simulink model "BuckBoost_real"  (R2015b)
settings: Solver=VariableStepAuto  StartTime=0.0  StopTime=0.01  RelTol=0.001
values from neighbouring files (symbols this model uses):
  Rload = 10    [BuckBoost_script.m]
libraries: fl_lib x7, elec_lib x5, nesl_utility x5
settings Model: Creator=lukaskiechle  LastModifiedBy=lukaskiechle
settings DataIOCC: LimitDataPoints=off  SaveFormat=Array
settings DebuggingCC: MaxConsecutiveZCsMsg=none
settings SimscapeCC: SimscapeLogType=all  SimscapeLogSimulationStatistics=on  SimscapeLogOpenViewer=on

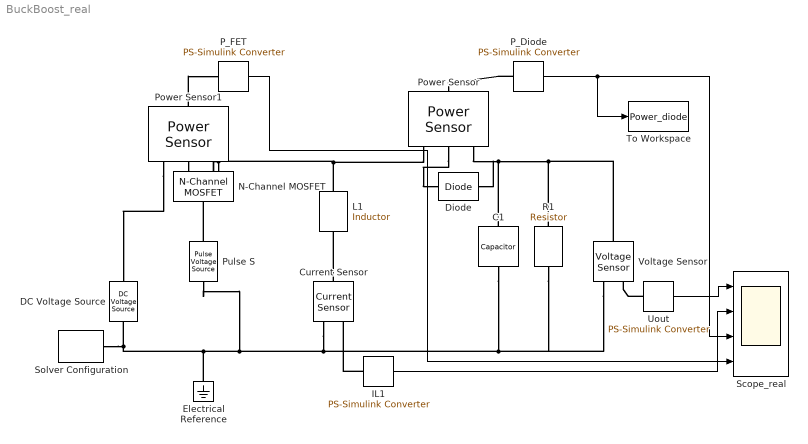
== system BuckBoost_real ==
  C1 : fl_lib/Electrical/Electrical Elements/Capacitor  c=C1 F  r=1e-9 Ohm  g=0 1/Ohm  i_specify=off  i_priority=None  i=0 A  v_specify=off  v_priority=None  v=0 V  vc_specify=off  vc_priority=None  vc=0 V
  Current Sensor : fl_lib/Electrical/Electrical Sensors/Current Sensor
  DC Voltage Source : fl_lib/Electrical/Electrical Sources/DC Voltage Source  v0=Uin V
  Diode : elec_lib/Semiconductor Devices/Diode  ModelType=2  Vf=UF V  Ron=0.08 Ohm  Goff=1E-9 S  Rz=0.1 Ohm  Vz=75 V  C_PWL=Diode_C F  prmExp=2  I12=[ 0.0137 0.545 ] A  V12=[ 0.6 0.7 ] V  I1=0.0137 A  V1=0.6 V  RS=0.01 Ohm  IS=1e-12 A  Tmeas=25 C  ec=1  BV=Inf V  C_param=1  CJ0=5 pF  VJ=1 V  Mgrad=0.5  Vvec=[ 0.1 10 100 ] V  Cvec=[ 3.5 1 0.4 ] pF  FC=0.5  Q_param=1  Irrm=-7.15 A  iF=4 A  didt=-750 A/us  trr=115 ns  TT=50 ns  tau=100 ns  T_param=1  IS_T2=1.25e-7 A  I1_T2=0.245 A  V1_T2=0.5 V  Tmeas2=125 C  EG_param=1  EG=1.11 eV  XTI_param=1  XTI=3  dBVdT=0 V/K  Tdevice=25 C  Rth=[ 0 10 ] K/W  thermal_mass_parameterization=1  thermal_mass=[ 0 1 ] J/K  thermal_time_constant=[ 0 10 ] s  thermal_mass_initial_temperatures=[ 25 25 ] C
  Electrical Reference : fl_lib/Electrical/Electrical Elements/Electrical Reference
  IL1 : nesl_utility/PS-Simulink Converter  PhysicalDomain=network_engine_domain  SubClassName=ps_output  LeftPortType=input  RightPortType=output  PseudoPeriodic=off  Frequencies=[]  Unit=A  AffineConversion=off
  L1 : fl_lib/Electrical/Electrical Elements/Inductor  l=L1 H  r=1 Ohm  g=1e-9 1/Ohm  i_specify=off  i_priority=None  i=0 A  v_specify=off  v_priority=None  v=0 V  i_L_specify=off  i_L_priority=None  i_L=0 A
  N-Channel MOSFET : elec_lib/Semiconductor Devices/N-Channel MOSFET  parameterization=1  prmDatasheet=1  prmEquCoeff=1  Beta=5 A/V^2  Rds=0.16 Ohm  Id=14 A  Vgs=10 V  Vth=3 V  lam=0 1/V  Tmeas=25 C  RS=1e-4 Ohm  RD=0.01 Ohm  C_param=1  C_GS=270 pF  C_GD=80 pF  C_iss=350 pF  C_rss=80 pF  C_oss=0 pF  C_GS_vec=[ 270 300 290 280 295 255 ] pF  C_GD_vec=[ 450 400 300 190 95 55 ] pF  C_iss_vec=[ 720 700 590 470 390 310 ] pF  C_rss_vec=[ 450 400 300 190 95 55 ] pF  C_oss_vec=[ 900 810 690 420 270 170 ] pF  C_Vds_vec=[ 0.1 0.3 1 3 10 30 ] V  charge_linearity_param=1  C_OX=200 pF  V_C_OX=-0.5 V  dVth_dT=-6 mV/K  Rds_T2=0.037 Ohm  Tmeas2=125 C  BEXDatasheet=-1.5  BEXEquCoeff=-1.5  TdeviceDatasheet=25 C  TdeviceEquCoeff=25 C  Rth=[ 0 10 ] K/W  thermal_mass_parameterization=1  thermal_mass=[ 0 1 ] J/K  thermal_time_constant=[ 0 10 ] s  thermal_mass_initial_temperatures=[ 25 25 ] C
  P_Diode : nesl_utility/PS-Simulink Converter  PhysicalDomain=network_engine_domain  SubClassName=ps_output  LeftPortType=input  RightPortType=output  PseudoPeriodic=off  Frequencies=[]  Unit=W  AffineConversion=off
  P_FET : nesl_utility/PS-Simulink Converter  PhysicalDomain=network_engine_domain  SubClassName=ps_output  LeftPortType=input  RightPortType=output  PseudoPeriodic=off  Frequencies=[]  Unit=W  AffineConversion=off
  Power Sensor : elec_lib/Sensors/Power Sensor  measurement_type=1  averaging_period=1 ms
  Power Sensor1 : elec_lib/Sensors/Power Sensor  measurement_type=1  averaging_period=1e-4 s
  Pulse S : elec_lib/Additional Components/SPICE-Compatible Components/Sources/Pulse Voltage Source  V1=0 V  V2=Upulse V  TD=0 s  TR=1e-9 s  TF=1e-9 s  PW=Ton s  PER=Twidth s
  R1 : fl_lib/Electrical/Electrical Elements/Resistor  R=Rload Ohm  i_specify=off  i_priority=None  i=0 A  v_specify=off  v_priority=None  v=0 V
  Scope_real : Scope  NumInputPorts=4
  Solver Configuration : nesl_utility/Solver Configuration  PhysicalDomain=network_engine_domain  SubClassName=solver  LeftPortType=input  RightPortType=generic  Accelerate=off  Tones=[]  Harmonics=[]  SimulateNoise=off  Profile=off  UseLocalSampling=off  EnableSwitchedLinearOptims=on  FrequencyDomain=off  UseCCode=off  RelTol=0.001  AbsTol=1e-06  MinStep=1e-09  ToWorkspace=off  RevertToSquareIcSolve=off  NumHomotopyIterations=100  PhasorMode=off  PhasorModeNumHarmonics=1  DoDC=off  ResidualTolerance=1e-09  UseLocalSolver=off  LocalSolverChoice=NE_BACKWARD_EULER_ADVANCER  LocalSolverSampleTime=0.001  DoFixedCost=off  MaxNonlinIter=3  MaxModeIter=2  LinearAlgebra=Sparse  DelaysMemoryBudget=1024  AutomaticFiltering=on  FilteringTimeConstant=0.001
  To Workspace : ToWorkspace  VariableName=Power_diode  SampleTime=-1
  Uout : nesl_utility/PS-Simulink Converter  PhysicalDomain=network_engine_domain  SubClassName=ps_output  LeftPortType=input  RightPortType=output  PseudoPeriodic=off  Frequencies=[]  Unit=V  AffineConversion=off
  Voltage Sensor : fl_lib/Electrical/Electrical Sensors/Voltage Sensor
  wires:
  Uout/1 -> Scope_real/1
  IL1/1 -> Scope_real/2
  P_Diode/1 -> To Workspace/1, Scope_real/3
  P_FET/1 -> Scope_real/4
  connections:
  Electrical Reference/LConn1 -- Pulse S/RConn1 -- Voltage Sensor/RConn2 -- R1/RConn1 -- C1/RConn1 -- Current Sensor/RConn2 -- Solver Configuration/RConn1 -- DC Voltage Source/RConn1
  Voltage Sensor/LConn1 -- Power Sensor/LConn3 -- Diode/LConn1 -- C1/LConn1 -- R1/LConn1
  Uout/LConn1 -- Voltage Sensor/RConn1
  Pulse S/LConn1 -- N-Channel MOSFET/LConn1
  Current Sensor/LConn1 -- L1/RConn1
  IL1/LConn1 -- Current Sensor/RConn1
  L1/LConn1 -- Power Sensor/LConn1 -- Power Sensor1/LConn3 -- N-Channel MOSFET/RConn2
  P_Diode/LConn1 -- Power Sensor/RConn1
  Power Sensor1/RConn1 -- P_FET/LConn1
  Power Sensor1/LConn1 -- DC Voltage Source/LConn1
  Power Sensor1/LConn2 -- N-Channel MOSFET/RConn1
  Power Sensor/LConn2 -- Diode/RConn1
